simulink model "Moving_Average_Filter"  (R2012b)
settings: Solver=ode45  StartTime=0.0  StopTime=10.0  RelTol=1e-3
settings Model: Creator=Ahmad  LastModifiedBy=Ahmad

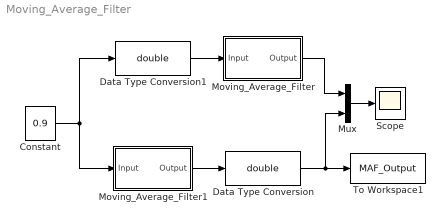
== system Moving_Average_Filter ==
  Constant : Constant  Value=0.9  VectorParams1D=off  OutDataTypeStr=fixdt(1,14,13)  SampleTime=1/50e6
  Data Type Conversion : DataTypeConversion  OutDataTypeStr=double
  Data Type Conversion1 : DataTypeConversion  OutDataTypeStr=double
  Moving_Average_Filter : Subsystem  Tag=FilterWizardSubSystem
      settings: ErrorFcn=dspFilterRealizedInBasicElemsAlgLoopErrFcnCallback
  Moving_Average_Filter1 : Subsystem  Tag=FilterWizardSubSystem
      settings: ErrorFcn=dspFilterRealizedInBasicElemsAlgLoopErrFcnCallback
  Mux : Mux  Inputs=2
  Scope : Scope
      settings: YMin=0.1  YMax=0.85
  To Workspace1 : ToWorkspace  VariableName=MAF_Output  SampleTime=-1  SaveFormat=Timeseries
  wires:
  Constant/1 -> Moving_Average_Filter1/1(Input), Data Type Conversion1/1
  Moving_Average_Filter1/1(Output) -> Data Type Conversion/1
  Data Type Conversion/1 -> Mux/2, To Workspace1/1
  Moving_Average_Filter/1(Output) -> Mux/1
  Mux/1 -> Scope/1
  Data Type Conversion1/1 -> Moving_Average_Filter/1(Input)

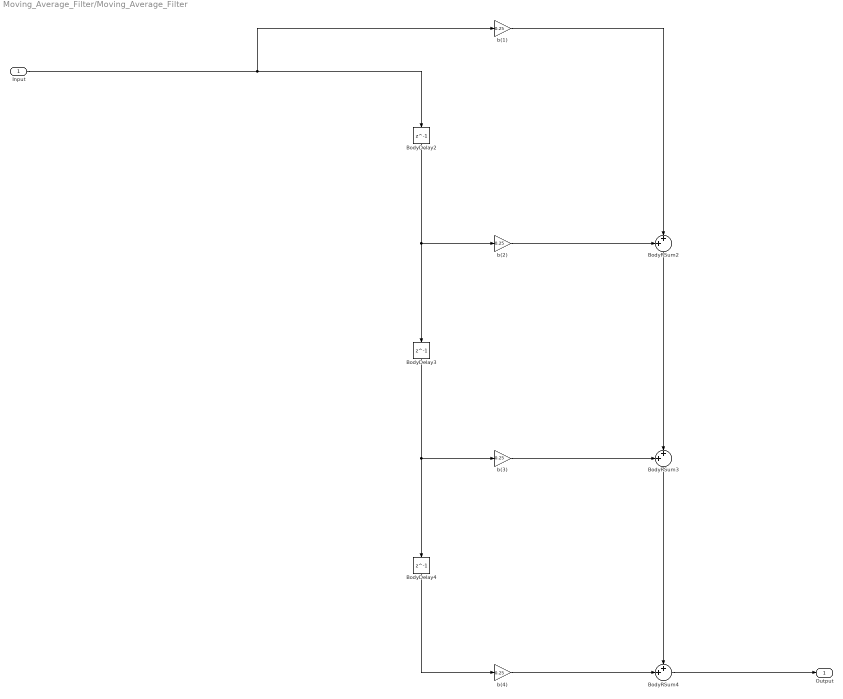
== system Moving_Average_Filter/Moving_Average_Filter ==
  Input : Inport
  BodyDelay2 : Delay  DelayLength=1  InitialCondition=0
  BodyDelay3 : Delay  DelayLength=1  InitialCondition=0
  BodyDelay4 : Delay  DelayLength=1  InitialCondition=0
  BodyRSum2 : Sum  Inputs=++|  RndMeth=Nearest  SaturateOnIntegerOverflow=on  OutDataTypeStr=Inherit: Same as first input
  BodyRSum3 : Sum  Inputs=++|  RndMeth=Nearest  SaturateOnIntegerOverflow=on  OutDataTypeStr=Inherit: Same as first input
  BodyRSum4 : Sum  Inputs=++|  RndMeth=Nearest  SaturateOnIntegerOverflow=on  OutDataTypeStr=Inherit: Same as first input
  b(1) : Gain  Gain=0.25  ParamDataTypeStr=double  RndMeth=Nearest  SaturateOnIntegerOverflow=on  OutDataTypeStr=Inherit: Same as input
  b(2) : Gain  Gain=0.25  ParamDataTypeStr=double  RndMeth=Nearest  SaturateOnIntegerOverflow=on  OutDataTypeStr=Inherit: Same as input
  b(3) : Gain  Gain=0.25  ParamDataTypeStr=double  RndMeth=Nearest  SaturateOnIntegerOverflow=on  OutDataTypeStr=Inherit: Same as input
  b(4) : Gain  Gain=0.25  ParamDataTypeStr=double  RndMeth=Nearest  SaturateOnIntegerOverflow=on  OutDataTypeStr=Inherit: Same as input
  Output : Outport
  wires:
  b(1)/1 -> BodyRSum2/2
  Input/1 -> b(1)/1, BodyDelay2/1
  BodyDelay2/1 -> b(2)/1, BodyDelay3/1
  b(2)/1 -> BodyRSum2/1
  BodyRSum2/1 -> BodyRSum3/2
  BodyDelay3/1 -> b(3)/1, BodyDelay4/1
  b(3)/1 -> BodyRSum3/1
  BodyRSum3/1 -> BodyRSum4/1
  BodyDelay4/1 -> b(4)/1
  b(4)/1 -> BodyRSum4/2
  BodyRSum4/1 -> Output/1

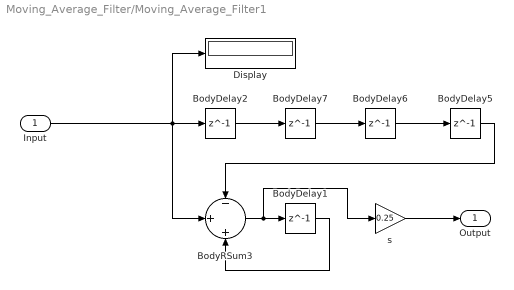
== system Moving_Average_Filter/Moving_Average_Filter1 ==
  Input : Inport
  BodyDelay{1..2,5..7} (5 alike) : Delay  DelayLength=1  InitialCondition=0
  BodyRSum3 : Sum  Inputs=-|+|+  AccumDataTypeStr=fixdt(1,16,13)  OutDataTypeStr=fixdt(1,16,13)  SaturateOnIntegerOverflow=on
  Display : Display
  s : Gain  Gain=0.25  ParamDataTypeStr=fixdt(1,3,2)  OutDataTypeStr=fixdt(1,14,13)  SaturateOnIntegerOverflow=on
  Output : Outport
  wires:
  BodyDelay2/1 -> BodyDelay7/1
  BodyDelay7/1 -> BodyDelay6/1
  BodyDelay6/1 -> BodyDelay5/1
  BodyDelay5/1 -> BodyRSum3/1
  BodyRSum3/1 -> s/1, BodyDelay1/1
  BodyDelay1/1 -> BodyRSum3/3
  s/1 -> Output/1
  Input/1 -> BodyRSum3/2, Display/1, BodyDelay2/1
